simulink model "que7"  (R2020b)
settings: Solver=VariableStepAuto  StartTime=0.0  StopTime=10.0  RelTol=1e-3
settings Model: Creator=hp  LastModifiedBy=hp

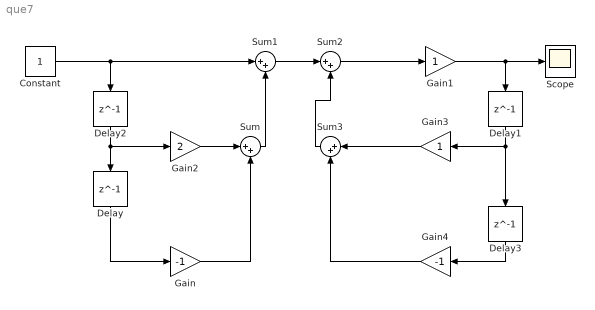
== system que7 ==
  Constant : Constant
  Delay{,1..3} (4 alike) : Delay  DelayLength=1  InitialCondition=0
  Gain : Gain  Gain=-1
  Gain1 : Gain
  Gain2 : Gain  Gain=2
  Gain3 : Gain
  Gain4 : Gain  Gain=-1
  Scope : Scope
  Sum{,1..3} (4 alike) : Sum  Inputs=|++
  wires:
  Delay/1 -> Gain/1
  Gain/1 -> Sum/2
  Sum/1 -> Sum1/2
  Gain2/1 -> Sum/1
  Delay2/1 -> Gain2/1, Delay/1
  Constant/1 -> Delay2/1, Sum1/1
  Sum1/1 -> Sum2/1
  Sum3/1 -> Sum2/2
  Sum2/1 -> Gain1/1
  Gain1/1 -> Scope/1, Delay1/1
  Gain3/1 -> Sum3/1
  Delay1/1 -> Delay3/1, Gain3/1
  Gain4/1 -> Sum3/2
  Delay3/1 -> Gain4/1
